simulink model "Parim_for_ai"  (R2024b)
settings: Solver=FixedStepDiscrete  StartTime=0.0  StopTime=3  FixedStep=Ts  RelTol=1e-3
PreLoadFcn:
  | Net_improve_init;L=Lac_MV;Tctrl=Ts;
PostLoadFcn:
  | Net_improve_init;L=Lac_MV;Tctrl=Ts;
InitFcn:
  | Net_improve_init;L=Lac_MV;Tctrl=Ts;
values from neighbouring files (symbols this model uses):
  Ts = 20e-6    (= 2e-05)    [Parsim_for_ai.m]
undefined symbols (not defined in the file or in its folder): C1, dend, DiscIntNeverNeededParam, fs, Lac_MV, numd, Pref, R1, Rac_MV, Vac_peak_MV, Vdc
libraries: powerlib_extras x10, spsControlledVoltageSourceLib x8, spsVoltageMeasurementLib x7, spsCurrentMeasurementLib x6, spsGroundLib x6, spsSeriesRLCBranchLib x6, spsACVoltageSourceLib x6, spsThreePhaseVIMeasurementLib x4, spsIdealSwitchLib x2, spsPower3phInstantaneousLib x2, simulink x2, spsThreePhaseSeriesRLCBranchLib x2
(part 1 of 2)
Description:
  | The Model initialization function Callback automatically
  | 
  | sets the sample time  to 2e-6 sec.  and loads the initial
  | 
  | states vector xInitial. The initial state vector is saved in the
  | 
  | power_acdrive_init.mat file.
  | 
  | 
  | 
  | Check  the Initial state checkbox in the Simulation
  | 
  | parameters/Workspace I/O to start in steady state with a
  | 
  | speed of 120 rad/s and a torque of 0 N.m/s,
  | 
  | 
  | Copyright 2008-2015 The MathWorks, Inc.
settings Model: Creator=WeiLi  LastModifiedBy=KeXing
settings SolverCC: AlgebraicLoopSolver=TrustRegion
settings DataIOCC: SaveFinalState=on  SaveFormat=Array  SignalLoggingSaveFormat=ModelDataLogs  SaveOutput=off  SaveTime=off  ReturnWorkspaceOutputs=off  SignalLoggingName=sigsOut
settings OptimizationCC: BlockReduction=off  ExpressionDepthLimit=2147483647  InitFltsAndDblsToZero=on  LifeSpan=inf
settings DebuggingCC: SaveWithParameterizedLinksMsg=none  UnderspecifiedInitializationDetection=Classic  MergeDetectMultiDrivingBlocksExec=none  CheckExecutionContextPreStartOutputMsg=on  SignalResolutionControl=TryResolveAllWithWarning  MultiTaskDSMMsg=warning  MultiTaskCondExecSysMsg=none  FcnCallInpInsideContextMsg=warning  UnconnectedInputMsg=warning  UnconnectedLineMsg=warning  StateNameClashWarn=warning  SFUnexpectedBacktrackingDiag=warning  SFNoUnconditionalDefaultTransitionDiag=warning  SFExecutionAtInitializationDiag=none  ArithmeticOperatorsInVariantConditions=warning
settings HardwareCC: ProdBitPerPointer=32  ProdBitPerSizeT=32  ProdBitPerPtrDiffT=32  ProdLargestAtomicFloat=None  ProdIntDivRoundTo=Undefined  ProdEndianess=Unspecified  ProdWordSize=32  ProdHWDeviceType=32-bit Generic  TargetUnknown=on
settings ModelReferenceCC: EnableRefExpFcnMdlSchedulingChecks=on  PropagateSignalLabelsOutOfModel=off
settings SFSimCC: SimUseLocalCustomCode=off  CustomCodeUndefinedFunction=UseInterfaceOnly
settings RTWCC: RTWUseLocalCustomCode=off  GPUComputeCapability=3.5
settings CodeAppCC: StateflowObjectComments=on
settings GRTTargetCC: TargetFcnLib=ansi_tfl_tmw.mat  TargetLangStandard=C89/C90 (ANSI)  CombineOutputUpdateFcns=off  GRTInterface=on
settings ConfigComp: CovMetricSettings=dw  CovSaveCumulativeToWorkspaceVar=on  CovSaveSingleToWorkspaceVar=on  CovExternalEMLEnable=off
settings SimscapeCC: SimscapeNormalizeSystem=off

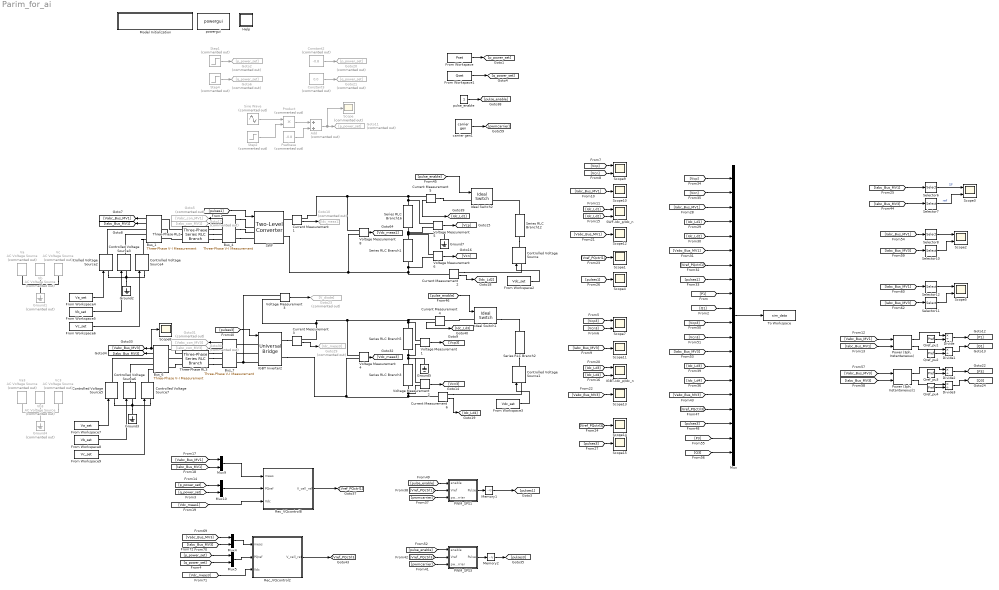
== system Parim_for_ai ==
  Add : Sum  Commented=on
  Bus_{1,4,6..7} (4 alike) : spsThreePhaseVIMeasurementLib/Three-Phase V-I Measurement  VoltageMeasurement=phase-to-ground  SetLabelV=off  LabelV=Vabc  Vpu=off  VpuLL=off  CurrentMeasurement=yes  SetLabelI=off  LabelI=Iabc  Ipu=off  Pbase=P_AC  Vbase=V_AC_prim  OutputType=Complex  PhasorSimulation=off  PSBequivalent=0
  Constant2 : Constant  Commented=on  Value=-0.8
  Constant3 : Constant  Commented=on  Value=0.0
  Controlled Voltage Source : spsControlledVoltageSourceLib/Controlled Voltage Source  Initialize=on  Source_Type=DC  Amplitude=3000  Phase=0  Frequency=0  Measurements=None
  Controlled Voltage Source1 : spsControlledVoltageSourceLib/Controlled Voltage Source  Initialize=on  Source_Type=DC  Amplitude=3000  Phase=0  Frequency=0  Measurements=None
  Controlled Voltage Source{2..7} (6 alike) : spsControlledVoltageSourceLib/Controlled Voltage Source  Initialize=off  Source_Type=AC  Amplitude=0  Phase=0  Frequency=fs  Measurements=None
  Current Measurement{1..6} (6 alike) : spsCurrentMeasurementLib/Current Measurement  PhasorSimulation=off  OutputType=Complex  PSBequivalent=0
  Divide{,1..3} (4 alike) : Product  Inputs=*/
  From Workspace : FromWorkspace  VariableName=Pset
  From Workspace1 : FromWorkspace  VariableName=Qset
  From Workspace2 : FromWorkspace  VariableName=Vdc_set  SampleTime=Ts
  From Workspace3 : FromWorkspace  VariableName=Vdc_set  SampleTime=Ts
  From Workspace4 : FromWorkspace  VariableName=Va_set  SampleTime=Ts
  From Workspace5 : FromWorkspace  VariableName=Vb_set  SampleTime=Ts
  From Workspace6 : FromWorkspace  VariableName=Vc_set  SampleTime=Ts
  From Workspace7 : FromWorkspace  VariableName=Va_set  SampleTime=Ts
  From Workspace8 : FromWorkspace  VariableName=Vb_set  SampleTime=Ts
  From Workspace9 : FromWorkspace  VariableName=Vc_set  SampleTime=Ts
  Goto10 : Goto  Commented=on  GotoTag=Idc_meas1
  Goto11 : Goto  Commented=on  GotoTag=p_power_set
  Goto17 : Goto  Commented=on  GotoTag=iabc_con_MV1
  Goto2 : Goto  Commented=on  GotoTag=p_power_set
  Goto20 : Goto  Commented=on  GotoTag=p_power_set
  Goto21 : Goto  Commented=on  GotoTag=q_power_set
  Goto23 : Goto  Commented=on  GotoTag=V_diode
  Goto29 : Goto  Commented=on  GotoTag=Idc_meas3
  Goto30 : Goto  Commented=on  GotoTag=iabc_con_MV3
  Goto31 : Goto  Commented=on  GotoTag=Vabc_con_MV3
  Goto5 : Goto  Commented=on  GotoTag=Vabc_con_MV1
  Goto6 : Goto  Commented=on  GotoTag=q_power_set
  Ground1 : spsGroundLib/Ground  Commented=on  LConnTagsString=a
  Ground{2..3,5,7} (4 alike) : spsGroundLib/Ground  LConnTagsString=a
  Ground4 : spsGroundLib/Ground  Commented=on  LConnTagsString=a
  Help : Subsystem  mask(OpDoc){docfile=../Help/help.html}
      mask init:
      | %patch([1,1,0,0,.8,1],[.8,0,0,1,1,.8],[.8 .8 .8]);
      | %patch([.15 .78 .78 .15 .15],[.8 .8 .83 .83 .8],[.9 .9 .9]);
      | %patch([.15 .78 .78 .15 .15],[.7 .7 .73 .73 .8],[.9 .9 .9]);
      | %patch([.15 .78 .78 .15 .15],[.6 .6 .63 .63 .6],[.9 .9 .9]);
      | %patch([.15 .78 .78 .15 .15],[.5 .5 .53 .53 .5],[.9 .9 .9]);
      | %patch([.15 .78 .78 .15 .15],[.4 .4 .43 .43 .4],[.9 .9 .9]);
      settings: OpenFcn=OpHelp_cb(gcb);
      mask Display: image(imread('opdoc.bmp'))
  IGBT Inverter2 : spsUniversalBridgeLib/Universal Bridge  Arms=3  SnubberResistance=IGBT_Rs  SnubberCapacitance=1e-6  Device=IGBT / Diodes  Ron=IGBT_Ron  Lon=0  ForwardVoltages=[0 0]  ForwardVoltage=.8  GTOparameters=[ 1e-6 , 1e-6 ]  IGBTparameters=[0 0]  Measurements=Device voltages  Measurements_2=None  converterType=Rectifier
      settings: AttributesFormatString=\n
  IGBT-Idc_p/Idc_n : Scope  NumInputPorts=2
  Ideal Switch1 : spsIdealSwitchLib/Ideal Switch  Ron=0.001  Lon=0  IC=0  Rs=1e9  Cs=inf  Measurements=on
  Ideal Switch2 : spsIdealSwitchLib/Ideal Switch  Ron=0.001  Lon=0  IC=0  Rs=1e9  Cs=inf  Measurements=on
  Memory1 : Memory
  Memory2 : Memory
  Model Initialization : Subsystem  mask(Model Functions){InitFcnX=Net_improve_init;L=Lac_MV;Tctrl=Ts;, prel=on, posl=on, inif=on, strf=off}
      mask prompts: InitFcnX "Initialisation"; prel "Preload Function"; posl "PostLoad Function"; inif "InitFcn"; strf "StartFcn"
      mask init:
      | currentBlock = gcb;
      | root = bdroot(currentBlock);
      | 
      | if ~strcmp(get_param(root,'BlockDiagramType'),'library')
      |     if prel==1
      |         set_param(root, 'PreLoadFcn', InitFcnX);
      |     else
      |         set_param(root, 'PreLoadFcn', '');
      |     end
      |     if inif==1
      |         set_param(root, 'InitFcn', InitFcnX);
      |     else
      |         set_param(root, 'InitFcn', '');
      |     end
      |     if strf==1
      |         set_param(root, 'StartFcn', InitFcnX);
      |     else
      |         set_param(root, 'StartFcn', '');
      |     end
      |     if posl==1
      |         set_param(root, 'PostLoadFcn', InitFcnX);
      |     else
      |         set_param(root, 'PostLoadFcn', '');
      |     end
      | end
      | 
      | pos = get_param(currentBlock, 'Position');
      | width = pos(3) - pos(1); height = pos(4) - pos(2);
      | txt = [ upper(root) '\n' '- InitFcn. . . . . '  get_param(root, 'InitFcn') ];
      settings: CopyFcn=set_param(gcb,'LinkStatus','none')
      mask Display: text(5, height*0.5, txt, 'horizontalAlignment', 'left', 'verticalAlignment', 'middle') ;
  Mux : Mux  Inputs=20
  Mux{4..5,9..10} (4 alike) : Mux  Inputs=2
  PWM_SPS1 : Subsystem
  PWM_SPS3 : Subsystem
  "Power (3ph, Instantaneous)" : spsPower3phInstantaneousLib/Power (3ph, Instantaneous)
  "Power (3ph, Instantaneous)1" : spsPower3phInstantaneousLib/Power (3ph, Instantaneous)
  Product : Product  Commented=on
  Psetbase : Constant  Commented=on  Value=-0.8
  Qref_pu{1..4} (4 alike) : Constant  Value=Pref
  Rec_VQcontrol2 : Subsystem  mask(converter controller){cm=off, base=[Pref, Vac_peak_MV*sqrt(3/2), Vdc/2, fs], LRx=[Lac_MV, Rac_MV], LRx_inpu=off, Kd=[0.3  2]*10/6  %was [1 0.1]   ; [0.1  1]*1, Kp=[0.3 1]*1     %was [1 0.1]   ; [0.1  1]*1, Kvdc=[2 10]*1;   %was [0.5 1]*20 for Cdc=320uF, Vabc_lim=[-1 1], limitVdq=1.1, nadv=6, xtrIctrl1=[0.4 10 10 -10], Ts=Tctrl}
      mask prompts: cm "control mode (check VQ/uncheck PQ), only one terminal in VQ mode"; base "base value for power(VA), ac voltage(V), dc voltage to ground(V), and frequenvy(Hz) [Sb, Vb, Vdcb,freq]"; LRx "commutation inductance and resistance [Lx, Rx]"; LRx_inpu "[Lx, Rx] in pu if checked/ SI unchecked"; Kd "Kp Ki for d-axis PI control [kp ki]"; Kp "Kp Ki for q-axis PI control [kp ki]"; Kvdc "Kp Ki for Vdc PI control [kp ki]"; Vabc_lim "output Vabc limit [min max]"; limitVdq "limit for Vd,Vq (pu, default = 1.1)"; nadv "nb of time step to compesate for delay (default=1)"; xtrIctrl1 "[kp, kp, limitmax, limitmin] for current control (default=[0.4, 10, 10, -10])"
      mask help:
      | input 1, 6 dimentions, Vabc, Iabc, (SI)
      | input 2, 2 dimentions, Pref, Qref (PU)
      | input 3, 6 dimentions, Vcap at up arm a, lower arm a, up arm b, lower arm b, up arm c and lower arm c.
      | input 4, 1 dimention, pulse on
      | input 5, 1 dimention
      |
      | power or current directions: to go into grid is positive
      mask init:
      | if cm==0;
      |     x=['PQ\nmode'];
      | else
      |     x=['VQ\nmode'];
      | end
      | 
      | Sb=base(1);            %VA 3phase power base;
      | Vb=base(2);       %V, line-line rms voltage base
      | Ib=Sb/(sqrt(3)*Vb); %A, rms current base
      | Zb=Vb^2/Sb ;        %ohm, impedence base
      | Vdc=base(3);      %V Vdc+ to ground or ground to Vdc- 
      | frq=base(4);
      | 
      | if LRx_inpu
      |     Rxpu=LRx(2);
      |     Lxpu=LRx(1);
      | else
      |     Rxpu=LRx(2)/Zb;
      |     Lxpu=LRx(1)*2*pi*frq/Zb;
      | end;
      | 
      | ks=Vdc*sqrt(3/2)/Vb;     % ma=1/ks for 1pu dc ->1pu ac;
      | 
      | Kp=Kd;
      mask DialogControl ParameterTabVar0 Prompt: parameters
      mask DialogControl ParameterTabVar01 Prompt: advanced
      mask Display: disp (x);
  Rec_VQcontrol8 : Subsystem  mask(converter controller){cm=off, base=[Pref, Vac_peak_MV*sqrt(3/2), Vdc/2, fs], LRx=[Lac_MV, Rac_MV], LRx_inpu=off, Kd=[0.3  2]*10/6  %was [1 0.1]   ; [0.1  1]*1, Kp=[0.3 1]*1     %was [1 0.1]   ; [0.1  1]*1, Kvdc=[2 10]*1;   %was [0.5 1]*20 for Cdc=320uF, Vabc_lim=[-1 1], limitVdq=1.1, nadv=6, xtrIctrl1=[0.4 10 10 -10], Ts=Tctrl}
      mask prompts: cm "control mode (check VQ/uncheck PQ), only one terminal in VQ mode"; base "base value for power(VA), ac voltage(V), dc voltage to ground(V), and frequenvy(Hz) [Sb, Vb, Vdcb,freq]"; LRx "commutation inductance and resistance [Lx, Rx]"; LRx_inpu "[Lx, Rx] in pu if checked/ SI unchecked"; Kd "Kp Ki for d-axis PI control [kp ki]"; Kp "Kp Ki for q-axis PI control [kp ki]"; Kvdc "Kp Ki for Vdc PI control [kp ki]"; Vabc_lim "output Vabc limit [min max]"; limitVdq "limit for Vd,Vq (pu, default = 1.1)"; nadv "nb of time step to compesate for delay (default=1)"; xtrIctrl1 "[kp, kp, limitmax, limitmin] for current control (default=[0.4, 10, 10, -10])"
      mask help:
      | input 1, 6 dimentions, Vabc, Iabc, (SI)
      | input 2, 2 dimentions, Pref, Qref (PU)
      | input 3, 6 dimentions, Vcap at up arm a, lower arm a, up arm b, lower arm b, up arm c and lower arm c.
      | input 4, 1 dimention, pulse on
      | input 5, 1 dimention
      |
      | power or current directions: to go into grid is positive
      mask init: same as Parim_for_ai/Rec_VQcontrol2
      mask DialogControl ParameterTabVar0 Prompt: parameters
      mask DialogControl ParameterTabVar01 Prompt: advanced
      mask Display: disp (x);
  SWF : spsTwoLevelConverterLib/Two-Level Converter  ModelType=Switching function  Ron=1e-3  Rs=1e6  Cs=inf  Vforward=[0,0]  Ron_Diode=IGBT_Ron  Rs_Diode=IGBT_Rs  Cs_Diode=1e-6  Vf_Diode=0  Rs_CurrentSource=inf  Ron_ACsource=1e-3
      settings: LibrarySourceBlock=sps_lib/Power Electronics/Two-Level Converter
  SWF-Idc_p/Idc_n : Scope  NumInputPorts=2
  Scope : Scope  Commented=on
  Scope{1,4,8,10..15} (9 alike) : Scope
  Scope{2..3,5,7,9} (5 alike) : Scope  NumInputPorts=2
  Selector10 : Selector  InputPortWidth=3  IndexOptions=Index vector (dialog)  Indices=[2]  OutputSizes=1
  Selector11 : Selector  InputPortWidth=3  IndexOptions=Index vector (dialog)  Indices=[3]  OutputSizes=1
  Selector12 : Selector  InputPortWidth=3  IndexOptions=Index vector (dialog)  Indices=[3]  OutputSizes=1
  Selector6 : Selector  InputPortWidth=3  IndexOptions=Index vector (dialog)  Indices=[1]  OutputSizes=1
  Selector7 : Selector  InputPortWidth=3  IndexOptions=Index vector (dialog)  Indices=[1]  OutputSizes=1
  Selector8 : Selector  InputPortWidth=3  IndexOptions=Index vector (dialog)  Indices=[2]  OutputSizes=1
  Series RLC Branch{1,3,5,16} (4 alike) : spsSeriesRLCBranchLib/Series RLC Branch  LConnTagsString=__new0  RConnTagsString=__new0  BranchType=C  Resistance=R1  Inductance=1e-3  SetiL0=off  InitialCurrent=0  Capacitance=C1  Setx0=off  InitialVoltage=0  Measurements=None
  Series RLC Branch12 : spsSeriesRLCBranchLib/Series RLC Branch  LConnTagsString=__new0  RConnTagsString=__new0  BranchType=R  Resistance=Vdc^2/(Pref)/10*2  Inductance=1e-3  SetiL0=off  InitialCurrent=0  Capacitance=C1  Setx0=off  InitialVoltage=0  Measurements=None
  Series RLC Branch2 : spsSeriesRLCBranchLib/Series RLC Branch  LConnTagsString=__new0  RConnTagsString=__new0  BranchType=R  Resistance=Vdc^2/(Pref)/10*2  Inductance=1e-3  SetiL0=off  InitialCurrent=0  Capacitance=C1  Setx0=off  InitialVoltage=0  Measurements=None
  Sine Wave : Sin  Commented=on  Amplitude=0.2  Frequency=20*2*pi  SampleTime=0
  Step1 : Step  Commented=on  Time=2  Before=-0.8  After=-0.5  SampleTime=0
  Step2 : Step  Commented=on  SampleTime=0
  Step4 : Step  Commented=on  Time=1.5  Before=0.0  After=0.0  SampleTime=0
  Three-Phase RL2 : spsThreePhaseSeriesRLCBranchLib/Three-Phase Series RLC Branch  LConnTagsString=A|B|C  RConnTagsString=A|B|C  BranchType=RL  Resistance=Rac_MV  Inductance=Lac_MV  Capacitance=1e-6  Measurements=None
  Three-Phase RL3 : spsThreePhaseSeriesRLCBranchLib/Three-Phase Series RLC Branch  LConnTagsString=A|B|C  RConnTagsString=A|B|C  BranchType=RL  Resistance=Rac_MV  Inductance=Lac_MV  Capacitance=1e-6  Measurements=None
  To Workspace : ToWorkspace  VariableName=sim_data  SampleTime=-1
      settings: Save2DSignal=2-D array (concatenate along first dimension)
  Va : spsACVoltageSourceLib/AC Voltage Source  Commented=on  Amplitude=Vac_peak_MV  Phase=0  Frequency=fs  SampleTime=Ts  Measurements=None  BusType=swing  Pref=10e3  Qref=0  Qmin=-inf  Qmax=+inf
  Va3 : spsACVoltageSourceLib/AC Voltage Source  Commented=on  Amplitude=Vac_peak_MV  Phase=0  Frequency=fs  SampleTime=Ts  Measurements=None  BusType=swing  Pref=10e3  Qref=0  Qmin=-inf  Qmax=+inf
  Vb : spsACVoltageSourceLib/AC Voltage Source  Commented=on  Amplitude=Vac_peak_MV  Phase=-120  Frequency=fs  SampleTime=Ts  Measurements=None  BusType=swing  Pref=10e3  Qref=0  Qmin=-inf  Qmax=+inf
  Vb3 : spsACVoltageSourceLib/AC Voltage Source  Commented=on  Amplitude=Vac_peak_MV  Phase=-120  Frequency=fs  SampleTime=Ts  Measurements=None  BusType=swing  Pref=10e3  Qref=0  Qmin=-inf  Qmax=+inf
  Vc : spsACVoltageSourceLib/AC Voltage Source  Commented=on  Amplitude=Vac_peak_MV  Phase=120  Frequency=fs  SampleTime=Ts  Measurements=None  BusType=swing  Pref=10e3  Qref=0  Qmin=-inf  Qmax=+inf
  Vc3 : spsACVoltageSourceLib/AC Voltage Source  Commented=on  Amplitude=Vac_peak_MV  Phase=120  Frequency=fs  SampleTime=Ts  Measurements=None  BusType=swing  Pref=10e3  Qref=0  Qmin=-inf  Qmax=+inf
  Voltage Measurement{1..6,8} (7 alike) : spsVoltageMeasurementLib/Voltage Measurement  PhasorSimulation=off  OutputType=Complex  PSBequivalent=0
  carrier gen1 : libMMCcpuv2/carrier gen  fc=f_cari  range=[ 1 -1]  Ms=3  Ns=1
  powergui : spspowerguiLib/powergui  Priority=2  SimulationMode=Discrete  SampleTime=Ts  frequency=60  Iterations=50  frequencyindice=0  Pbase=100e6  ErrMax=1e-4  UnitsV=kV  UnitsW=MW  buscounter=0  FunctionMessages=off  echomessages=off  EnableUseOfTLC=off  CurrentSourceSwitches=off  DisableSnubberDevices=off  DisableRonSwitches=off  DisableVfSwitches=off  DisplayEquations=off  AutomaticDiscreteSolvers=off  SolverType=Backward Euler  Interpol=off  ExternalGateDelay=off  methode=off  Ts=0  x0status=blocks  SPID=off  SwTol=0  HookPort=off  NonlinearTolerance=1e-4  nMaxIteration=100  ContinueOnMaxIteration=off  RestoreLinks=warning  ResistiveCurrentMeasurement=off  Frange=[0:2:500]  Ylog=off  Xlog=on  ShowGrid=off  save=off  variable=ZData  structure=VI  ZoomFFT=off  StartTime=9  cycles=10  DisplayStyle=2  fundamental=300/pi  FreqAxis=off  MaxFrequency=1000  frequencyindicesteady=1  RmsSteady=1  display=off
  pulse_enable : Constant
  wires:
  Bus_1/1 -> [Vabc_Bus_MV1]
  Bus_1/2 -> [Iabc_Bus_MV1]
  Bus_4/1 -> Goto5/1
  Current Measurement1/1 -> Goto10/1
  [Vabc_Bus_MV1] -> Mux9/1
  [Iabc_Bus_MV1] -> Mux9/2
  [q_power_set] -> Mux10/2
  carrier gen1/1 -> [pwmcarrier]
  [p_power_set] -> Mux10/1
  [pwmcarrier] -> PWM_SPS1/3(pwmcarrier)
  [Vref_PQctrl1] -> PWM_SPS1/2(Vref)
  Mux9/1 -> Rec_VQcontrol8/1(meas)
  Mux10/1 -> Rec_VQcontrol8/2(PQref)
  [Vdc_meas1] -> Rec_VQcontrol8/3(Vdc)
  Voltage Measurement8/1 -> [Vdc_meas1]
  Bus_4/2 -> Goto17/1
  [Iabc_Bus_MV1] -> Selector6/1
  Step2/1 -> Product/2
  Voltage Measurement3/1 -> Goto23/1
  Bus_6/1 -> Scope8/1, [Vabc_Bus_MV3]
  Bus_6/2 -> [Iabc_Bus_MV3]
  Bus_7/1 -> Goto31/1
  Current Measurement3/1 -> Goto29/1
  Voltage Measurement4/1 -> [Vdc_meas3]
  Bus_7/2 -> Goto30/1
  [pwmcarrier] -> PWM_SPS3/3(pwmcarrier)
  [Vref_PQctrl3] -> PWM_SPS3/2(Vref)
  [Iabc_Bus_MV3] -> Selector7/1
  [pulse_enable] -> PWM_SPS1/1(enable)
  [pulse_enable] -> PWM_SPS3/1(enable)
  Current Measurement5/1 -> [Idc_Ld1]
  Current Measurement4/1 -> [Idc_Ld3]
  [pulses3] -> IGBT Inverter2/1
  Selector6/1 -> Scope3/1  "SF"
  Selector7/1 -> Scope3/2  "ref"
  [Iabc_Bus_MV1] -> Selector8/1
  [Iabc_Bus_MV3] -> Selector10/1
  Selector8/1 -> Scope2/1
  Selector10/1 -> Scope2/2
  [Iabc_Bus_MV1] -> Selector12/1
  [Iabc_Bus_MV3] -> Selector11/1
  Selector12/1 -> Scope5/1
  Selector11/1 -> Scope5/2
  PWM_SPS1/1(Pulse) -> Memory1/1
  [Vabc_Bus_MV3] -> Mux4/1
  [Iabc_Bus_MV3] -> Mux4/2
  Mux4/1 -> Rec_VQcontrol2/1(meas)
  Mux5/1 -> Rec_VQcontrol2/2(PQref)
  [q_power_set] -> Mux5/2
  [Vdc_meas3] -> Rec_VQcontrol2/3(Vdc)
  [p_power_set] -> Mux5/1
  [pulse_enable] -> Ideal Switch2/1
  [pulse_enable] -> Ideal Switch1/1
  Memory1/1 -> [pulses1]
  pulse_enable/1 -> [pulse_enable]
  PWM_SPS3/1(Pulse) -> Memory2/1
  Rec_VQcontrol8/1(V_cell_ref) -> [Vref_PQctrl1]
  Rec_VQcontrol2/1(V_cell_ref) -> [Vref_PQctrl3]
  Memory2/1 -> [pulses3]
  "Power (3ph, Instantaneous)"/1 -> Divide/1
  Qref_pu2/1 -> Divide1/2
  [Iabc_Bus_MV1] -> "Power (3ph, Instantaneous)"/2
  Divide1/1 -> [Q1]
  Qref_pu1/1 -> Divide/2
  Divide/1 -> [P1]
  [Vabc_Bus_MV1] -> "Power (3ph, Instantaneous)"/1
  "Power (3ph, Instantaneous)"/2 -> Divide1/1
  From Workspace1/1 -> [q_power_set]
  Step1/1 -> Goto2/1
  Product/1 -> Add/1
  Psetbase/1 -> Add/2
  Add/1 -> Scope/1, Goto11/1
  Sine Wave/1 -> Product/1
  From Workspace/1 -> [p_power_set]
  Step4/1 -> Goto6/1
  Voltage Measurement1/1 -> [Vcp3]
  Voltage Measurement2/1 -> [Vcn3]
  [Vcp3] -> Scope7/1
  [Vcn3] -> Scope7/2
  Voltage Measurement5/1 -> [Vcp]
  Voltage Measurement6/1 -> [Vcn]
  [Vcp] -> Scope9/1
  [Vcn] -> Scope9/2
  [Iabc_Bus_MV1] -> Scope10/1
  [Iabc_Bus_MV3] -> Scope11/1
  Current Measurement2/1 -> [Idc_Ld2]
  Current Measurement6/1 -> [Idc_Ld4]
  [Idc_Ld1] -> SWF-Idc_p/Idc_n/1
  [Idc_Ld2] -> SWF-Idc_p/Idc_n/2
  [Idc_Ld3] -> IGBT-Idc_p/Idc_n/1
  [Idc_Ld4] -> IGBT-Idc_p/Idc_n/2
  [Vabc_Bus_MV1] -> Scope12/1
  [Vabc_Bus_MV3] -> Scope13/1
  [Vref_PQctrl1] -> Scope1/1
  [pulses1] -> Scope4/1
  [Vref_PQctrl3] -> Scope14/1
  [pulses3] -> Scope15/1
  Constant2/1 -> Goto20/1
  Constant3/1 -> Goto21/1
  [Vcp] -> Mux/1
  [Vcn] -> Mux/2
  [Iabc_Bus_MV1] -> Mux/3
  [Idc_Ld1] -> Mux/4
  [Idc_Ld2] -> Mux/5
  [Vabc_Bus_MV1] -> Mux/6
  [Vref_PQctrl1] -> Mux/7
  [pulses1] -> Mux/8
  Mux/1 -> To Workspace/1
  From Workspace2/1 -> Controlled Voltage Source/1
  From Workspace3/1 -> Controlled Voltage Source1/1
  [P1] -> Mux/9
  [Q1] -> Mux/10
  [pulses3] -> Mux/18
  [Iabc_Bus_MV3] -> Mux/13
  [Idc_Ld4] -> Mux/15
  [Vcp3] -> Mux/11
  [Idc_Ld3] -> Mux/14
  [Vref_PQctrl3] -> Mux/17
  [Vcn3] -> Mux/12
  [Vabc_Bus_MV3] -> Mux/16
  "Power (3ph, Instantaneous)1"/1 -> Divide2/1
  Qref_pu3/1 -> Divide2/2
  Divide3/1 -> [Q3]
  "Power (3ph, Instantaneous)1"/2 -> Divide3/1
  Qref_pu4/1 -> Divide3/2
  Divide2/1 -> [P3]
  [Iabc_Bus_MV3] -> "Power (3ph, Instantaneous)1"/2
  [Vabc_Bus_MV3] -> "Power (3ph, Instantaneous)1"/1
  [Q3] -> Mux/20
  [P3] -> Mux/19
  From Workspace4/1 -> Controlled Voltage Source2/1
  From Workspace5/1 -> Controlled Voltage Source3/1
  From Workspace6/1 -> Controlled Voltage Source4/1
  [pulses1] -> SWF/1
  From Workspace7/1 -> Controlled Voltage Source5/1
  From Workspace8/1 -> Controlled Voltage Source6/1
  From Workspace9/1 -> Controlled Voltage Source7/1
  connections:
  Three-Phase RL2/LConn1 -- Bus_1/LConn1
  Three-Phase RL2/LConn3 -- Bus_1/LConn3
  Three-Phase RL2/LConn2 -- Bus_1/LConn2
  Three-Phase RL2/RConn1 -- Bus_4/RConn1
  Three-Phase RL2/RConn2 -- Bus_4/RConn2
  Three-Phase RL2/RConn3 -- Bus_4/RConn3
  Series RLC Branch1/RConn1 -- Voltage Measurement6/LConn2 -- Current Measurement2/LConn1 -- Voltage Measurement8/LConn2 -- SWF/RConn2
  Voltage Measurement8/LConn1 -- Current Measurement5/RConn1 -- Voltage Measurement5/LConn1 -- Series RLC Branch16/LConn1 -- Current Measurement1/RConn1
  Series RLC Branch1/LConn1 -- Voltage Measurement6/LConn1 -- Ground7/LConn1 -- Voltage Measurement5/LConn2 -- Series RLC Branch16/RConn1
  IGBT Inverter2/LConn1 -- Bus_7/LConn1
  Series RLC Branch3/RConn1 -- Voltage Measurement2/LConn2 -- Current Measurement6/LConn1 -- IGBT Inverter2/RConn2 -- Voltage Measurement4/LConn2
  Series RLC Branch5/LConn1 -- Voltage Measurement1/LConn1 -- Current Measurement4/RConn1 -- Voltage Measurement4/LConn1 -- Voltage Measurement3/LConn2 -- Current Measurement3/RConn1
  Series RLC Branch3/LConn1 -- Voltage Measurement2/LConn1 -- Ground5/LConn1 -- Voltage Measurement1/LConn2 -- Series RLC Branch5/RConn1
  IGBT Inverter2/RConn1 -- Current Measurement3/LConn1
  Three-Phase RL3/RConn1 -- Bus_7/RConn1
  Bus_6/RConn2 -- Controlled Voltage Source6/RConn1
  Three-Phase RL3/LConn2 -- Bus_6/LConn2
  Bus_6/RConn3 -- Controlled Voltage Source7/RConn1
  Three-Phase RL3/RConn3 -- Bus_7/RConn3
  Three-Phase RL3/RConn2 -- Bus_7/RConn2
  Three-Phase RL3/LConn3 -- Bus_6/LConn3
  Bus_6/RConn1 -- Controlled Voltage Source5/RConn1
  Three-Phase RL3/LConn1 -- Bus_6/LConn1
  IGBT Inverter2/LConn3 -- Voltage Measurement3/LConn1 -- Bus_7/LConn3
  IGBT Inverter2/LConn2 -- Bus_7/LConn2
  Ideal Switch1/RConn1 -- Series RLC Branch2/RConn1
  Current Measurement5/LConn1 -- Ideal Switch2/LConn1
  Series RLC Branch2/LConn1 -- Controlled Voltage Source1/RConn1
  Series RLC Branch12/LConn1 -- Controlled Voltage Source/RConn1
  Series RLC Branch12/RConn1 -- Ideal Switch2/RConn1
  Current Measurement2/RConn1 -- Controlled Voltage Source/LConn1
  Current Measurement6/RConn1 -- Controlled Voltage Source1/LConn1
  Vb3/LConn1 -- Vc3/LConn1 -- Va3/LConn1 -- Ground4/LConn1
  Ground1/LConn1 -- Vb/LConn1 -- Vc/LConn1 -- Va/LConn1
  Ground2/LConn1 -- Controlled Voltage Source4/LConn1 -- Controlled Voltage Source2/LConn1 -- Controlled Voltage Source3/LConn1
  Ground3/LConn1 -- Controlled Voltage Source7/LConn1 -- Controlled Voltage Source5/LConn1 -- Controlled Voltage Source6/LConn1
  Ideal Switch1/LConn1 -- Current Measurement4/LConn1
  Bus_1/RConn1 -- Controlled Voltage Source2/RConn1
  Bus_1/RConn2 -- Controlled Voltage Source3/RConn1
  Bus_1/RConn3 -- Controlled Voltage Source4/RConn1
  Current Measurement1/LConn1 -- SWF/RConn1
  Bus_4/LConn3 -- SWF/LConn3
  Bus_4/LConn2 -- SWF/LConn2
  Bus_4/LConn1 -- SWF/LConn1

== system Parim_for_ai/Help ==

== system Parim_for_ai/Model Initialization ==

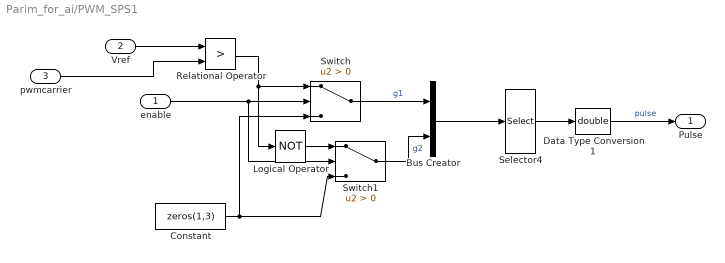
== system Parim_for_ai/PWM_SPS1 ==
  enable : Inport
  Vref : Inport  Port=2
  pwmcarrier : Inport  Port=3
  Bus Creator : BusCreator  Inputs=2
  Constant : Constant  Value=zeros(1,3)
  Data Type Conversion1 : DataTypeConversion  OutDataTypeStr=double  SaturateOnIntegerOverflow=off  RndMeth=Floor
  Logical Operator : Logic  Operator=NOT  AllPortsSameDT=off  OutDataTypeStr=boolean
  Relational Operator : RelationalOperator  Operator=>  OutDataTypeStr=boolean  InputSameDT=off
  Selector4 : Selector  InputPortWidth=6  IndexOptions=Index vector (dialog)  Indices=[1 4 2 5 3 6]  OutputSizes=1
  Switch : Switch  Criteria=u2 > Threshold  SaturateOnIntegerOverflow=off  InputSameDT=off
  Switch1 : Switch  Criteria=u2 > Threshold  SaturateOnIntegerOverflow=off  InputSameDT=off
  Pulse : Outport  VectorParamsAs1DForOutWhenUnconnected=off
  wires:
  Vref/1 -> Relational Operator/1
  pwmcarrier/1 -> Relational Operator/2
  enable/1 -> Switch1/2, Switch/2
  Relational Operator/1 -> Logical Operator/1, Switch/1
  Switch/1 -> Bus Creator/1  "g1"
  Switch1/1 -> Bus Creator/2  "g2"
  Logical Operator/1 -> Switch1/1
  Constant/1 -> Switch/3, Switch1/3
  Selector4/1 -> Data Type Conversion1/1
  Bus Creator/1 -> Selector4/1
  Data Type Conversion1/1 -> Pulse/1  "pulse"

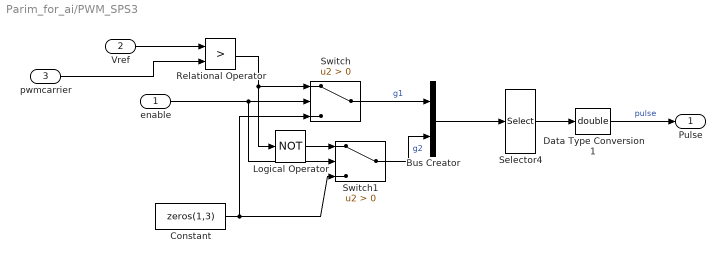
== system Parim_for_ai/PWM_SPS3 ==
  enable : Inport
  Vref : Inport  Port=2
  pwmcarrier : Inport  Port=3
  Bus Creator : BusCreator  Inputs=2
  Constant : Constant  Value=zeros(1,3)
  Data Type Conversion1 : DataTypeConversion  OutDataTypeStr=double  SaturateOnIntegerOverflow=off  RndMeth=Floor
  Logical Operator : Logic  Operator=NOT  AllPortsSameDT=off  OutDataTypeStr=boolean
  Relational Operator : RelationalOperator  Operator=>  OutDataTypeStr=boolean  InputSameDT=off
  Selector4 : Selector  InputPortWidth=6  IndexOptions=Index vector (dialog)  Indices=[1 4 2 5 3 6]  OutputSizes=1
  Switch : Switch  Criteria=u2 > Threshold  SaturateOnIntegerOverflow=off  InputSameDT=off
  Switch1 : Switch  Criteria=u2 > Threshold  SaturateOnIntegerOverflow=off  InputSameDT=off
  Pulse : Outport  VectorParamsAs1DForOutWhenUnconnected=off
  wires:
  Data Type Conversion1/1 -> Pulse/1  "pulse"
  Bus Creator/1 -> Selector4/1
  Selector4/1 -> Data Type Conversion1/1
  Constant/1 -> Switch1/3, Switch/3
  Logical Operator/1 -> Switch1/1
  Switch1/1 -> Bus Creator/2  "g2"
  Switch/1 -> Bus Creator/1  "g1"
  Relational Operator/1 -> Switch/1, Logical Operator/1
  enable/1 -> Switch/2, Switch1/2
  pwmcarrier/1 -> Relational Operator/2
  Vref/1 -> Relational Operator/1

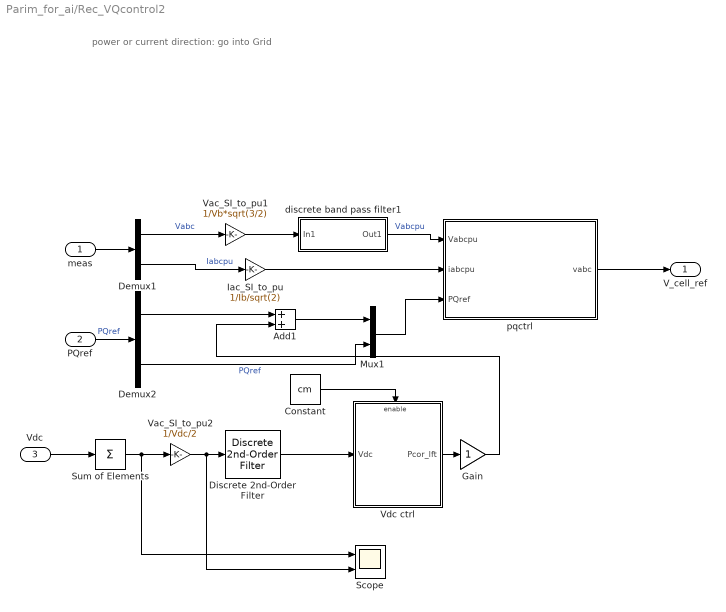
== system Parim_for_ai/Rec_VQcontrol2 ==
  note: power or current direction: go into Grid
  meas : Inport
  PQref : Inport  Port=2
  Vdc : Inport  Port=3
  Add1 : Sum
  Constant : Constant  Value=cm
  Demux1 : Demux  Outputs=[3 3 ]
  Demux2 : Demux  Outputs=2
  Discrete 2nd-Order Filter : powerlib_extras/Discrete  Control Blocks/Discrete  2nd-Order Filter  FilterType=Lowpass  Fo=90  Zeta=0.707  Ts=Ts  Initialize=off  Vac_Init=[0.8 -25 60]  Vdc_Init=-0.4  PlotResponse=off  param1=[1 500 1]
  Gain : Gain
  Iac_SI_to_pu : Gain  Gain=1/Ib/sqrt(2)
  Mux1 : Mux  Inputs=2
  Scope : Scope  NumInputPorts=2
  Sum of Elements : Sum  Inputs=+
  Vac_SI_to_pu1 : Gain  Gain=1/Vb*sqrt(3/2)
  Vac_SI_to_pu2 : Gain  Gain=1/Vdc/2  SampleTime=Ts
  Vdc ctrl : Subsystem
  discrete band pass filter1 : Subsystem  mask(discrete transfer Fcn generator){Fo=frq, adj1=1, inistate=0, Ts=Ts, bodedw=off}
      mask prompts: Fo "F0 (Hz)"; adj1 "adj (1 for no adjustment, larger adj for wider band pass)"; inistate "Initial states"; Ts "Sample time (must be explicite)"; bodedw "draw Bode diagram of filter"
      mask help:
      | This block transfer a continous TF to a discrete TF
      | using Bilinear (Tustin) approximation
      mask init:
      | AD1=tf([1 0],1);
      | 
      | %second order
      | % Fo=50; %cut off freq.
      | % omega0=Fo*2*pi;
      | % adj1=3;   %adjustment 1
      | Zeta= 0.707*adj1; %Damping factor Zeta ( Q = 1 / (2*Zeta) ):
      | Wo=2*pi*Fo;
      | % str=sprintf(' Fo=%iHz\n\n',Fo);
      |  n2=0; n1=0;n0=Wo*Wo;
      |  d2=1;d1=2*Zeta*Wo;d0=Wo*Wo;
      | numc=[n2 n1 n0];
      | denc=[d2 d1 d0];
      | AD3=tf(numc,denc);
      | 
      | AD4=AD1*AD3;
      | [mag1,pha1]=bode(AD4,Wo);
      | mag0=mag1;
      | AD=AD4/mag0;
      | 
      | if bodedw==1
      |     figure;
      |     h=bodeplot(AD1,AD3,AD);
      |     setoptions(h,'FreqUnits','Hz');
      |     grid on;
      |     title(['Bode Diagram, adj=',num2str(adj1)]);
      | end;
      |     
      | % gg=tf(num,den);
      | ggd=c2d(AD,Ts,'tustin');
      | [numd,dend] = tfdata(ggd,'v');
  pqctrl : Subsystem
  V_cell_ref : Outport  VectorParamsAs1DForOutWhenUnconnected=off
  wires:
  Gain/1 -> Add1/2
  Sum of Elements/1 -> Vac_SI_to_pu2/1, Scope/1
  pqctrl/1(vabc) -> V_cell_ref/1
  PQref/1 -> Demux2/1  "PQref"
  discrete band pass filter1/1(Out1) -> pqctrl/1(Vabcpu)  "Vabcpu"
  meas/1 -> Demux1/1
  Demux1/2 -> Iac_SI_to_pu/1  "Iabcpu"
  Demux1/1 -> Vac_SI_to_pu1/1  "Vabc"
  Iac_SI_to_pu/1 -> pqctrl/2(iabcpu)
  Demux2/1 -> Add1/1
  Vdc ctrl/1(Pcor_lft) -> Gain/1
  Add1/1 -> Mux1/1
  Demux2/2 -> Mux1/2  "PQref"
  Mux1/1 -> pqctrl/3(PQref)
  Discrete 2nd-Order Filter/1 -> Vdc ctrl/1(Vdc)
  Vdc/1 -> Sum of Elements/1
  Vac_SI_to_pu2/1 -> Discrete 2nd-Order Filter/1, Scope/2
  Vac_SI_to_pu1/1 -> discrete band pass filter1/1(In1)
  Constant/1 -> Vdc ctrl/Enable

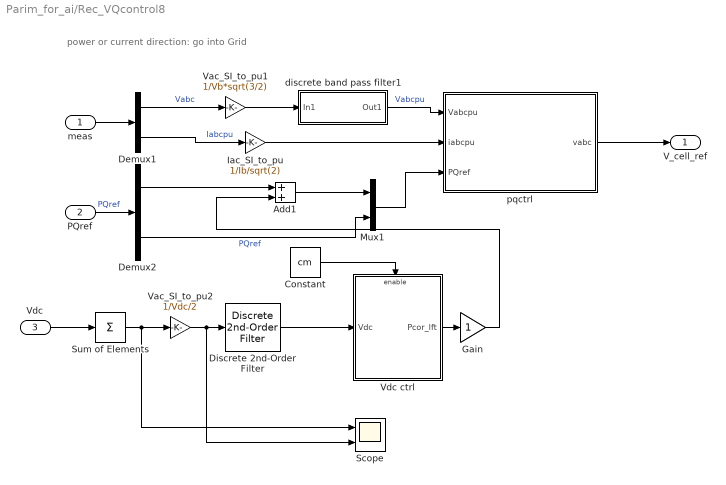
== system Parim_for_ai/Rec_VQcontrol8 ==
  note: power or current direction: go into Grid
  meas : Inport
  PQref : Inport  Port=2
  Vdc : Inport  Port=3
  Add1 : Sum
  Constant : Constant  Value=cm
  Demux1 : Demux  Outputs=[3 3 ]
  Demux2 : Demux  Outputs=2
  Discrete 2nd-Order Filter : powerlib_extras/Discrete  Control Blocks/Discrete  2nd-Order Filter  FilterType=Lowpass  Fo=90  Zeta=0.707  Ts=Ts  Initialize=off  Vac_Init=[0.8 -25 60]  Vdc_Init=-0.4  PlotResponse=off  param1=[1 500 1]
  Gain : Gain
  Iac_SI_to_pu : Gain  Gain=1/Ib/sqrt(2)
  Mux1 : Mux  Inputs=2
  Scope : Scope  NumInputPorts=2
  Sum of Elements : Sum  Inputs=+
  Vac_SI_to_pu1 : Gain  Gain=1/Vb*sqrt(3/2)
  Vac_SI_to_pu2 : Gain  Gain=1/Vdc/2  SampleTime=Ts
  Vdc ctrl : Subsystem
  discrete band pass filter1 : Subsystem  mask(discrete transfer Fcn generator){Fo=frq, adj1=1, inistate=0, Ts=Ts, bodedw=off}
      mask prompts: Fo "F0 (Hz)"; adj1 "adj (1 for no adjustment, larger adj for wider band pass)"; inistate "Initial states"; Ts "Sample time (must be explicite)"; bodedw "draw Bode diagram of filter"
      mask help:
      | This block transfer a continous TF to a discrete TF
      | using Bilinear (Tustin) approximation
      mask init: same as Parim_for_ai/Rec_VQcontrol2/discrete band pass filter1
  pqctrl : Subsystem
  V_cell_ref : Outport  VectorParamsAs1DForOutWhenUnconnected=off
  wires:
  Constant/1 -> Vdc ctrl/Enable
  Vac_SI_to_pu1/1 -> discrete band pass filter1/1(In1)
  Vac_SI_to_pu2/1 -> Scope/2, Discrete 2nd-Order Filter/1
  Vdc/1 -> Sum of Elements/1
  Discrete 2nd-Order Filter/1 -> Vdc ctrl/1(Vdc)
  Mux1/1 -> pqctrl/3(PQref)
  Demux2/2 -> Mux1/2  "PQref"
  Add1/1 -> Mux1/1
  Vdc ctrl/1(Pcor_lft) -> Gain/1
  Demux2/1 -> Add1/1
  Iac_SI_to_pu/1 -> pqctrl/2(iabcpu)
  Demux1/1 -> Vac_SI_to_pu1/1  "Vabc"
  Demux1/2 -> Iac_SI_to_pu/1  "Iabcpu"
  meas/1 -> Demux1/1
  discrete band pass filter1/1(Out1) -> pqctrl/1(Vabcpu)  "Vabcpu"
  PQref/1 -> Demux2/1  "PQref"
  pqctrl/1(vabc) -> V_cell_ref/1
  Sum of Elements/1 -> Scope/1, Vac_SI_to_pu2/1
  Gain/1 -> Add1/2

== system Parim_for_ai/Rec_VQcontrol2/Vdc ctrl ==
  Vdc : Inport
  Enable : EnablePort  StatesWhenEnabling=reset
  Vdc_ctrler1 : Subsystem
  Pcor_lft : Outport  OutputWhenDisabled=reset  InitialOutput=0  VectorParamsAs1DForOutWhenUnconnected=off
  wires:
  Vdc/1 -> Vdc_ctrler1/1(Vcap)
  Vdc_ctrler1/1(delP) -> Pcor_lft/1  "Pclft"

== system Parim_for_ai/Rec_VQcontrol2/discrete band pass filter1 ==
  In1 : Inport
  Discrete Transfer Fcn : DiscreteTransferFcn  Numerator=numd  Denominator=dend  InitialStates=inistate  SampleTime=Ts
  Out1 : Outport  VectorParamsAs1DForOutWhenUnconnected=off
  wires:
  In1/1 -> Discrete Transfer Fcn/1
  Discrete Transfer Fcn/1 -> Out1/1

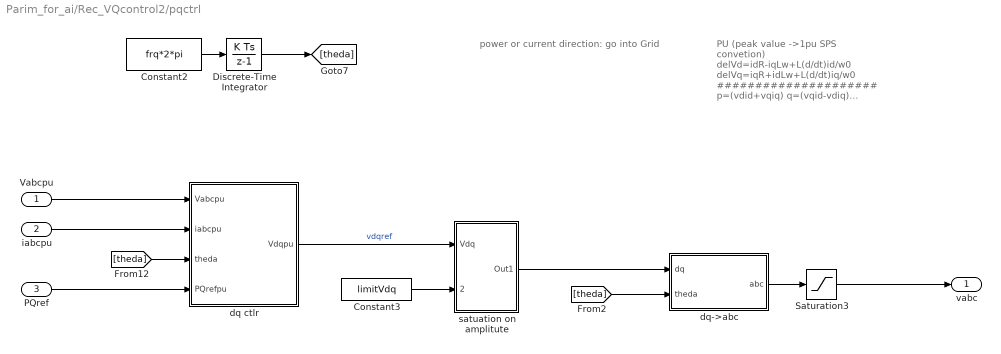
== system Parim_for_ai/Rec_VQcontrol2/pqctrl ==
  note: power or current direction: go into Grid
  note: PU
      | (peak value ->1pu
      | SPS convetion)
      |
      | delVd=idR-iqLw+L(d/dt)id/w0
      | delVq=iqR+idLw+L(d/dt)iq/w0
      | #####################
      | p=(vdid+vqiq)
      | q=(vqid-vdiq)
      | =>
      | Id=(Vd*P+Vq*Q)/C
      | Iq=(Vq*P-Vd*Q)/C
      | C=Vd^2+Vq^2
  Vabcpu : Inport
  iabcpu : Inport  Port=2
  PQref : Inport  Port=3
  Constant2 : Constant  Value=frq*2*pi
  Constant3 : Constant  Value=limitVdq
  Discrete-Time Integrator : DiscreteIntegrator  SampleTime=Ts  ICPrevOutput=DiscIntNeverNeededParam  ICPrevScaledInput=DiscIntNeverNeededParam
  Saturation3 : Saturate  UpperLimit=Vabc_lim(2)  LowerLimit=Vabc_lim(1)
  dq ctlr : Subsystem
  dq->abc : Subsystem
  "satuation on amplitute " : Subsystem
  vabc : Outport  VectorParamsAs1DForOutWhenUnconnected=off
  wires:
  PQref/1 -> dq ctlr/4(PQrefpu)
  iabcpu/1 -> dq ctlr/2(iabcpu)
  Vabcpu/1 -> dq ctlr/1(Vabcpu)
  dq ctlr/1(Vdqpu) -> "satuation on amplitute "/1(Vdq)  "vdqref"
  [theda] -> dq ctlr/3(theda)
  Discrete-Time Integrator/1 -> [theda]
  Constant2/1 -> Discrete-Time Integrator/1
  "satuation on amplitute "/1(Out1) -> dq->abc/1(dq)
  Constant3/1 -> "satuation on amplitute "/2(limitVdq)
  dq->abc/1(abc) -> Saturation3/1
  [theda] -> dq->abc/2(theda)
  Saturation3/1 -> vabc/1

== system Parim_for_ai/Rec_VQcontrol8/Vdc ctrl ==
  Vdc : Inport
  Enable : EnablePort  StatesWhenEnabling=reset
  Vdc_ctrler1 : Subsystem
  Pcor_lft : Outport  OutputWhenDisabled=reset  InitialOutput=0  VectorParamsAs1DForOutWhenUnconnected=off
  wires:
  Vdc_ctrler1/1(delP) -> Pcor_lft/1  "Pclft"
  Vdc/1 -> Vdc_ctrler1/1(Vcap)

== system Parim_for_ai/Rec_VQcontrol8/discrete band pass filter1 ==
  In1 : Inport
  Discrete Transfer Fcn : DiscreteTransferFcn  Numerator=numd  Denominator=dend  InitialStates=inistate  SampleTime=Ts
  Out1 : Outport  VectorParamsAs1DForOutWhenUnconnected=off
  wires:
  Discrete Transfer Fcn/1 -> Out1/1
  In1/1 -> Discrete Transfer Fcn/1

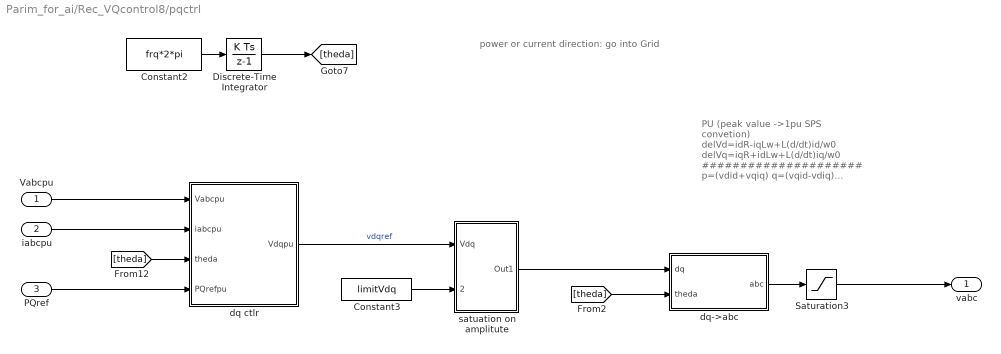
== system Parim_for_ai/Rec_VQcontrol8/pqctrl ==
  note: PU
      | (peak value ->1pu
      | SPS convetion)
      |
      | delVd=idR-iqLw+L(d/dt)id/w0
      | delVq=iqR+idLw+L(d/dt)iq/w0
      | #####################
      | p=(vdid+vqiq)
      | q=(vqid-vdiq)
      | =>
      | Id=(Vd*P+Vq*Q)/C
      | Iq=(Vq*P-Vd*Q)/C
      | C=Vd^2+Vq^2
  note: power or current direction: go into Grid
  Vabcpu : Inport
  iabcpu : Inport  Port=2
  PQref : Inport  Port=3
  Constant2 : Constant  Value=frq*2*pi
  Constant3 : Constant  Value=limitVdq
  Discrete-Time Integrator : DiscreteIntegrator  SampleTime=Ts  ICPrevOutput=DiscIntNeverNeededParam  ICPrevScaledInput=DiscIntNeverNeededParam
  Saturation3 : Saturate  UpperLimit=Vabc_lim(2)  LowerLimit=Vabc_lim(1)
  dq ctlr : Subsystem
  dq->abc : Subsystem
  "satuation on amplitute " : Subsystem
  vabc : Outport  VectorParamsAs1DForOutWhenUnconnected=off
  wires:
  Saturation3/1 -> vabc/1
  [theda] -> dq->abc/2(theda)
  dq->abc/1(abc) -> Saturation3/1
  Constant3/1 -> "satuation on amplitute "/2(limitVdq)
  "satuation on amplitute "/1(Out1) -> dq->abc/1(dq)
  Constant2/1 -> Discrete-Time Integrator/1
  Discrete-Time Integrator/1 -> [theda]
  [theda] -> dq ctlr/3(theda)
  dq ctlr/1(Vdqpu) -> "satuation on amplitute "/1(Vdq)  "vdqref"
  Vabcpu/1 -> dq ctlr/1(Vabcpu)
  iabcpu/1 -> dq ctlr/2(iabcpu)
  PQref/1 -> dq ctlr/4(PQrefpu)

== system Parim_for_ai/Rec_VQcontrol2/Vdc ctrl/Vdc_ctrler1 ==
  Vcap : Inport
  Add2 : Sum  Inputs=+-
  PI_d2 : Subsystem  AncestorBlock=|  DialogController=POWERSYS.PowerSysDialog  mask(Discrete PI Controller){Kp=Kvdc(1), Ki=Kvdc(2), Par_Limits=[1 -1]*1, Init=0, Ts=Ts}
      | powerlib_extras/Discrete 
      | Control Blocks/Discrete
      | PI Controller
      mask prompts: Kp "Proportional gain (Kp):"; Ki "Integral gain (Ki):"; Par_Limits "Output limits: [ Upper   Lower ]"; Init "Output initial value:"; Ts "Sample time:"
      mask help: This block implements a discrete PI controller.
      mask init:
      | UpperLimit=Par_Limits(1);
      | LowerLimit=Par_Limits(2);
      | power_initmask();
      mask Help: This block is part of a subset of blocks in the Extras library that does not have documentation associated with it, other than the block mask description.
      mask Display: disp('PI');
  Saturation : Saturate  UpperLimit=0.1  LowerLimit=-0.1
      settings: AttributesFormatString=%<LowerLimit>~%<UpperLimit>
  Vdcpuref : Constant
  Vdctrl : Scope  NumInputPorts=2
  delP : Outport  OutputWhenDisabled=reset  InitialOutput=[0]  VectorParamsAs1DForOutWhenUnconnected=off
  wires:
  Add2/1 -> Saturation/1  "delVdc"
  Vcap/1 -> Vdctrl/1, Add2/1
  Vdcpuref/1 -> Add2/2
  Saturation/1 -> PI_d2/1(Error)
  PI_d2/1(Out) -> Vdctrl/2, delP/1  "PIVdc"

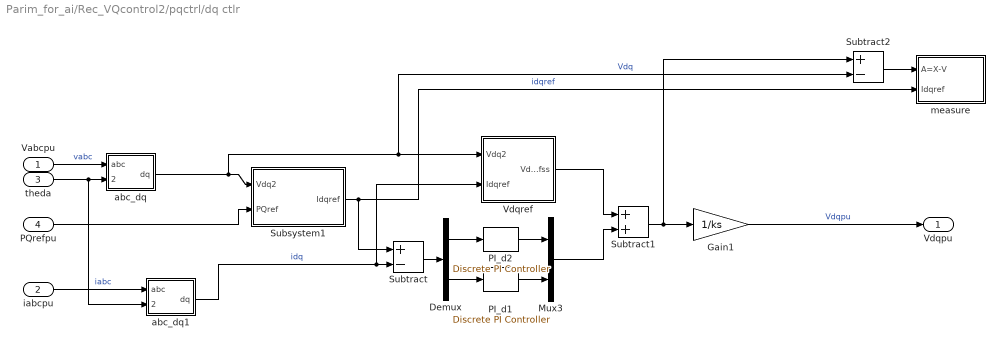
== system Parim_for_ai/Rec_VQcontrol2/pqctrl/dq ctlr ==
  Vabcpu : Inport
  iabcpu : Inport  Port=2
  theda : Inport  Port=3
  PQrefpu : Inport  Port=4
  Demux : Demux  Outputs=2
  Gain1 : Gain  Gain=1/ks
  Mux3 : Mux  Inputs=2
  PI_d1 : powerlib_extras/Discrete  Control Blocks/Discrete PI Controller  Kp=Kp(1)  Ki=Kp(2)  Par_Limits=[1 -1]*0.15  Init=0  Ts=Ts
  PI_d2 : powerlib_extras/Discrete  Control Blocks/Discrete PI Controller  Kp=Kd(1)  Ki=Kd(2)  Par_Limits=[1 -1]*0.25  Init=0  Ts=Ts
  Subsystem1 : Subsystem
  Subtract : Sum  Inputs=+-
  Subtract1 : Sum
  Subtract2 : Sum  Inputs=+-
  Vdqref : Subsystem
  abc_dq : Subsystem
  abc_dq1 : Subsystem
  measure : Subsystem
  Vdqpu : Outport  VectorParamsAs1DForOutWhenUnconnected=off
  wires:
  Gain1/1 -> Vdqpu/1  "Vdqpu"
  iabcpu/1 -> abc_dq1/1(abc)  "iabc"
  PQrefpu/1 -> Subsystem1/2(PQref)
  theda/1 -> abc_dq1/2(theta), abc_dq/2(theta)
  Vabcpu/1 -> abc_dq/1(abc)  "vabc"
  Subtract1/1 -> Gain1/1, Subtract2/1
  Mux3/1 -> Subtract1/2
  PI_d1/1 -> Mux3/2
  PI_d2/1 -> Mux3/1
  Vdqref/1(Vdqrefss) -> Subtract1/1
  Demux/2 -> PI_d1/1
  Demux/1 -> PI_d2/1
  Subtract/1 -> Demux/1
  abc_dq1/1(dq) -> Subtract/2, Vdqref/2(Idqref)  "idq"
  abc_dq/1(dq) -> Subsystem1/1(Vdq2), Vdqref/1(Vdq2), Subtract2/2  "Vdq"
  Subsystem1/1(Idqref) -> Subtract/1, measure/2(Idqref)  "idqref"
  Subtract2/1 -> measure/1(A=X-V)

== system Parim_for_ai/Rec_VQcontrol2/pqctrl/dq->abc ==
  note: Vc= Vd*sin(wt+2pi/3) + Vq*cos(wt+2pi/3) + Vo
  note: Vb= Vd*sin(wt-2pi/3) + Vq*cos(wt-2pi/3) + Vo
  note: Va= Vd*sinwt + Vq*cos(wt) + Vo
  dq : Inport
  theda : Inport  Port=2
  Fcn : Fcn  Expr=(u(1)*sin(u(3))+u(2)*cos(u(3)))
  Fcn1 : Fcn  Expr=(u(1)*sin(u(3)-2*pi/3)+u(2)*cos(u(3)-2*pi/3))
  Fcn2 : Fcn  Expr=(u(1)*sin(u(3)+2*pi/3)+u(2)*cos(u(3)+2*pi/3))
  Mux1 : Mux  Inputs=2
  Mux3 : Mux  Inputs=3
  abc : Outport  VectorParamsAs1DForOutWhenUnconnected=off
  wires:
  Mux3/1 -> abc/1  "abc"
  theda/1 -> Mux1/2
  dq/1 -> Mux1/1
  Mux1/1 -> Fcn1/1, Fcn2/1, Fcn/1
  Fcn/1 -> Mux3/1
  Fcn1/1 -> Mux3/2
  Fcn2/1 -> Mux3/3

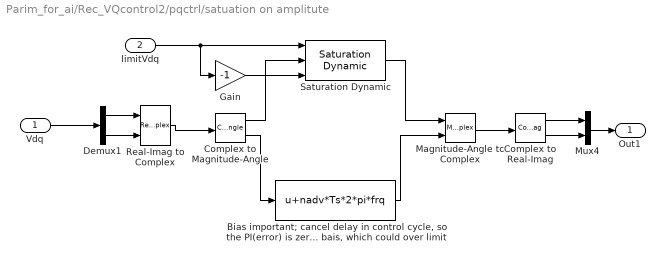
== system Parim_for_ai/Rec_VQcontrol2/pqctrl/satuation on amplitute  ==
  Vdq : Inport
  limitVdq : Inport  Port=2
  "Bias important; cancel delay in control cycle, so the PI(error) is zero, other wise PI(errer) is bais, which could over limit" : Bias  Bias=nadv*Ts*2*pi*frq  SaturateOnIntegerOverflow=off
  Complex to Magnitude-Angle : ComplexToMagnitudeAngle
  Complex to Real-Imag : ComplexToRealImag
  Demux1 : Demux  Outputs=2
  Gain : Gain  Gain=-1
  Magnitude-Angle to Complex : MagnitudeAngleToComplex
  Mux4 : Mux  Inputs=2
  Real-Imag to Complex : RealImagToComplex
  Saturation Dynamic : simulink/Discontinuities/Saturation Dynamic  OutMin=[]  OutMax=[]  OutDataTypeStr=Inherit: Same as second input  OutDataType=fixdt(1, 16)  OutScaling=2^-10  DoSatur=off
  Out1 : Outport  VectorParamsAs1DForOutWhenUnconnected=off
  wires:
  Vdq/1 -> Demux1/1
  Mux4/1 -> Out1/1
  Complex to Real-Imag/1 -> Mux4/1
  Complex to Real-Imag/2 -> Mux4/2
  Magnitude-Angle to Complex/1 -> Complex to Real-Imag/1
  Complex to Magnitude-Angle/2 -> "Bias important; cancel delay in control cycle, so the PI(error) is zero, other wise PI(errer) is bais, which could over limit"/1
  Real-Imag to Complex/1 -> Complex to Magnitude-Angle/1
  Demux1/2 -> Real-Imag to Complex/2
  Demux1/1 -> Real-Imag to Complex/1
  Saturation Dynamic/1 -> Magnitude-Angle to Complex/1
  Complex to Magnitude-Angle/1 -> Saturation Dynamic/2
  limitVdq/1 -> Gain/1, Saturation Dynamic/1
  Gain/1 -> Saturation Dynamic/3
  "Bias important; cancel delay in control cycle, so the PI(error) is zero, other wise PI(errer) is bais, which could over limit"/1 -> Magnitude-Angle to Complex/2

== system Parim_for_ai/Rec_VQcontrol8/Vdc ctrl/Vdc_ctrler1 ==
  Vcap : Inport
  Add2 : Sum  Inputs=+-
  PI_d2 : Subsystem  AncestorBlock=|  DialogController=POWERSYS.PowerSysDialog  mask(Discrete PI Controller){Kp=Kvdc(1), Ki=Kvdc(2), Par_Limits=[1 -1]*1, Init=0, Ts=Ts}
      | powerlib_extras/Discrete 
      | Control Blocks/Discrete
      | PI Controller
      mask prompts: Kp "Proportional gain (Kp):"; Ki "Integral gain (Ki):"; Par_Limits "Output limits: [ Upper   Lower ]"; Init "Output initial value:"; Ts "Sample time:"
      mask help: This block implements a discrete PI controller.
      mask init:
      | UpperLimit=Par_Limits(1);
      | LowerLimit=Par_Limits(2);
      | power_initmask();
      mask Help: This block is part of a subset of blocks in the Extras library that does not have documentation associated with it, other than the block mask description.
      mask Display: disp('PI');
  Saturation : Saturate  UpperLimit=0.1  LowerLimit=-0.1
      settings: AttributesFormatString=%<LowerLimit>~%<UpperLimit>
  Vdcpuref : Constant
  Vdctrl : Scope  NumInputPorts=2
  delP : Outport  OutputWhenDisabled=reset  InitialOutput=[0]  VectorParamsAs1DForOutWhenUnconnected=off
  wires:
  PI_d2/1(Out) -> delP/1, Vdctrl/2  "PIVdc"
  Saturation/1 -> PI_d2/1(Error)
  Vdcpuref/1 -> Add2/2
  Vcap/1 -> Add2/1, Vdctrl/1
  Add2/1 -> Saturation/1  "delVdc"

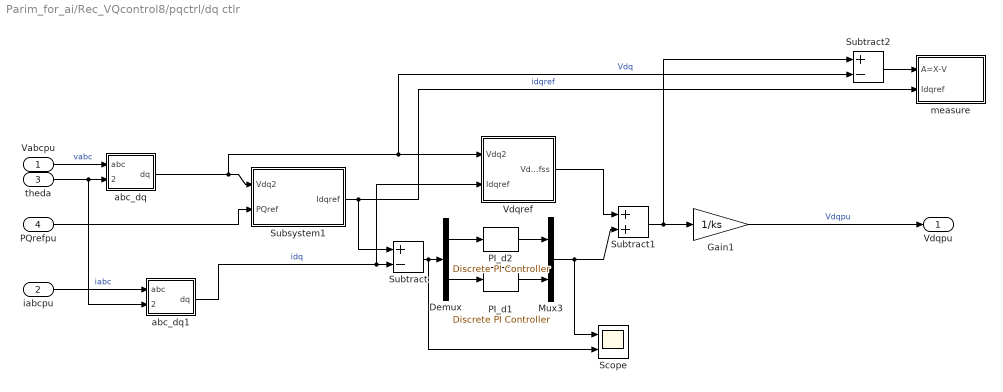
== system Parim_for_ai/Rec_VQcontrol8/pqctrl/dq ctlr ==
  Vabcpu : Inport
  iabcpu : Inport  Port=2
  theda : Inport  Port=3
  PQrefpu : Inport  Port=4
  Demux : Demux  Outputs=2
  Gain1 : Gain  Gain=1/ks
  Mux3 : Mux  Inputs=2
  PI_d1 : powerlib_extras/Discrete  Control Blocks/Discrete PI Controller  Kp=Kp(1)  Ki=Kp(2)  Par_Limits=[1 -1]*0.15  Init=0  Ts=Ts
  PI_d2 : powerlib_extras/Discrete  Control Blocks/Discrete PI Controller  Kp=Kd(1)  Ki=Kd(2)  Par_Limits=[1 -1]*0.25  Init=0  Ts=Ts
  Scope : Scope  NumInputPorts=2
  Subsystem1 : Subsystem
  Subtract : Sum  Inputs=+-
  Subtract1 : Sum
  Subtract2 : Sum  Inputs=+-
  Vdqref : Subsystem
  abc_dq : Subsystem
  abc_dq1 : Subsystem
  measure : Subsystem
  Vdqpu : Outport  VectorParamsAs1DForOutWhenUnconnected=off
  wires:
  Subtract2/1 -> measure/1(A=X-V)
  Subsystem1/1(Idqref) -> measure/2(Idqref), Subtract/1  "idqref"
  abc_dq/1(dq) -> Subtract2/2, Vdqref/1(Vdq2), Subsystem1/1(Vdq2)  "Vdq"
  abc_dq1/1(dq) -> Vdqref/2(Idqref), Subtract/2  "idq"
  Subtract/1 -> Scope/2, Demux/1
  Demux/1 -> PI_d2/1
  Demux/2 -> PI_d1/1
  Vdqref/1(Vdqrefss) -> Subtract1/1
  PI_d2/1 -> Mux3/1
  PI_d1/1 -> Mux3/2
  Mux3/1 -> Scope/1, Subtract1/2
  Subtract1/1 -> Subtract2/1, Gain1/1
  Vabcpu/1 -> abc_dq/1(abc)  "vabc"
  theda/1 -> abc_dq/2(theta), abc_dq1/2(theta)
  PQrefpu/1 -> Subsystem1/2(PQref)
  iabcpu/1 -> abc_dq1/1(abc)  "iabc"
  Gain1/1 -> Vdqpu/1  "Vdqpu"

== system Parim_for_ai/Rec_VQcontrol8/pqctrl/dq->abc ==
  note: Va= Vd*sinwt + Vq*cos(wt) + Vo
  note: Vb= Vd*sin(wt-2pi/3) + Vq*cos(wt-2pi/3) + Vo
  note: Vc= Vd*sin(wt+2pi/3) + Vq*cos(wt+2pi/3) + Vo
  dq : Inport
  theda : Inport  Port=2
  Fcn : Fcn  Expr=(u(1)*sin(u(3))+u(2)*cos(u(3)))
  Fcn1 : Fcn  Expr=(u(1)*sin(u(3)-2*pi/3)+u(2)*cos(u(3)-2*pi/3))
  Fcn2 : Fcn  Expr=(u(1)*sin(u(3)+2*pi/3)+u(2)*cos(u(3)+2*pi/3))
  Mux1 : Mux  Inputs=2
  Mux3 : Mux  Inputs=3
  abc : Outport  VectorParamsAs1DForOutWhenUnconnected=off
  wires:
  Fcn2/1 -> Mux3/3
  Fcn1/1 -> Mux3/2
  Fcn/1 -> Mux3/1
  Mux1/1 -> Fcn/1, Fcn2/1, Fcn1/1
  dq/1 -> Mux1/1
  theda/1 -> Mux1/2
  Mux3/1 -> abc/1  "abc"

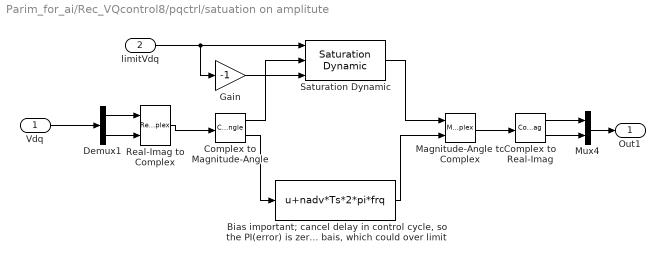
== system Parim_for_ai/Rec_VQcontrol8/pqctrl/satuation on amplitute  ==
  Vdq : Inport
  limitVdq : Inport  Port=2
  "Bias important; cancel delay in control cycle, so the PI(error) is zero, other wise PI(errer) is bais, which could over limit" : Bias  Bias=nadv*Ts*2*pi*frq  SaturateOnIntegerOverflow=off
  Complex to Magnitude-Angle : ComplexToMagnitudeAngle
  Complex to Real-Imag : ComplexToRealImag
  Demux1 : Demux  Outputs=2
  Gain : Gain  Gain=-1
  Magnitude-Angle to Complex : MagnitudeAngleToComplex
  Mux4 : Mux  Inputs=2
  Real-Imag to Complex : RealImagToComplex
  Saturation Dynamic : simulink/Discontinuities/Saturation Dynamic  OutMin=[]  OutMax=[]  OutDataTypeStr=Inherit: Same as second input  OutDataType=fixdt(1, 16)  OutScaling=2^-10  DoSatur=off
  Out1 : Outport  VectorParamsAs1DForOutWhenUnconnected=off
  wires:
  "Bias important; cancel delay in control cycle, so the PI(error) is zero, other wise PI(errer) is bais, which could over limit"/1 -> Magnitude-Angle to Complex/2
  Gain/1 -> Saturation Dynamic/3
  limitVdq/1 -> Saturation Dynamic/1, Gain/1
  Complex to Magnitude-Angle/1 -> Saturation Dynamic/2
  Saturation Dynamic/1 -> Magnitude-Angle to Complex/1
  Demux1/1 -> Real-Imag to Complex/1
  Demux1/2 -> Real-Imag to Complex/2
  Real-Imag to Complex/1 -> Complex to Magnitude-Angle/1
  Complex to Magnitude-Angle/2 -> "Bias important; cancel delay in control cycle, so the PI(error) is zero, other wise PI(errer) is bais, which could over limit"/1
  Magnitude-Angle to Complex/1 -> Complex to Real-Imag/1
  Complex to Real-Imag/2 -> Mux4/2
  Complex to Real-Imag/1 -> Mux4/1
  Mux4/1 -> Out1/1
  Vdq/1 -> Demux1/1

== system Parim_for_ai/Rec_VQcontrol2/Vdc ctrl/Vdc_ctrler1/PI_d2 ==
  note: Pierre Giroux, Gilbert Sybille
      | Power System Simulation Laboratory
      | IREQ, Hydro-Quebc
  note: Discrete PID Controller
  Error : Inport  SampleTime=Ts
  Discrete-Time Integrator : DiscreteIntegrator  InitialCondition=Init  SampleTime=Ts  LimitOutput=on  UpperSaturationLimit=UpperLimit  LowerSaturationLimit=LowerLimit  ICPrevOutput=DiscIntNeverNeededParam  ICPrevScaledInput=DiscIntNeverNeededParam
  Kp4 : Gain  Gain=Kp  SaturateOnIntegerOverflow=on  SampleTime=Ts  OutDataTypeStr=Inherit: Same as input  ParamDataTypeStr=Inherit: Same as input
  Kp5 : Gain  Gain=Ki  SaturateOnIntegerOverflow=on  SampleTime=Ts  OutDataTypeStr=Inherit: Same as input  ParamDataTypeStr=Inherit: Same as input
  Saturation2 : Saturate  UpperLimit=UpperLimit  LowerLimit=LowerLimit  SampleTime=Ts
  Sum6 : Sum  InputSameDT=on  SaturateOnIntegerOverflow=on  SampleTime=Ts  OutDataTypeStr=Inherit: Same as first input
  Zero-Order Hold : ZeroOrderHold  SampleTime=Ts
  Out : Outport  SampleTime=Ts  InitialOutput=0  VectorParamsAs1DForOutWhenUnconnected=off
  wires:
  Error/1 -> Kp4/1, Kp5/1
  Sum6/1 -> Saturation2/1
  Kp5/1 -> Discrete-Time Integrator/1
  Kp4/1 -> Zero-Order Hold/1
  Discrete-Time Integrator/1 -> Sum6/2  "int"
  Saturation2/1 -> Out/1
  Zero-Order Hold/1 -> Sum6/1  "prop"

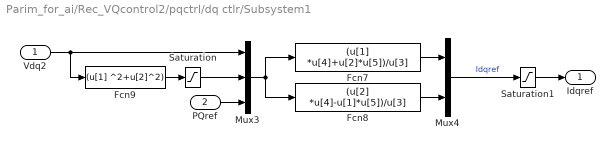
== system Parim_for_ai/Rec_VQcontrol2/pqctrl/dq ctlr/Subsystem1 ==
  Vdq2 : Inport
  PQref : Inport  Port=2
  Fcn7 : Fcn  Expr=(u[1] *u[4]+u[2]*u[5])/u[3]
  Fcn8 : Fcn  Expr=(u[2] *u[4]-u[1]*u[5])/u[3]
  Fcn9 : Fcn  Expr=(u[1] ^2+u[2]^2)
  Mux3 : Mux  Inputs=[2 1 2]
  Mux4 : Mux  Inputs=2
  Saturation : Saturate  UpperLimit=inf  LowerLimit=0.01
  Saturation1 : Saturate  UpperLimit=1.5  LowerLimit=-1.5
  Idqref : Outport  VectorParamsAs1DForOutWhenUnconnected=off
  wires:
  Saturation/1 -> Mux3/2
  PQref/1 -> Mux3/3
  Mux4/1 -> Saturation1/1  "Idqref"
  Fcn8/1 -> Mux4/2
  Fcn7/1 -> Mux4/1
  Fcn9/1 -> Saturation/1
  Mux3/1 -> Fcn7/1, Fcn8/1
  Vdq2/1 -> Mux3/1, Fcn9/1
  Saturation1/1 -> Idqref/1

== system Parim_for_ai/Rec_VQcontrol2/pqctrl/dq ctlr/Vdqref ==
  Vdq2 : Inport
  Idqref : Inport  Port=2
  Display : Display
      settings: Decimation=50
  Fcn7 : Fcn  Expr=(u[2] +u[4]*u[5]+u[3]*u[6])
  Fcn8 : Fcn  Expr=(u[1] +u[3]*u[5]-u[4]*u[6])
  Lxpu : Constant  Value=Lxpu
  Mux3 : Mux
  Mux4 : Mux  Inputs=2
  Rxpu : Constant  Value=Rxpu
  Vdqrefss : Outport  VectorParamsAs1DForOutWhenUnconnected=off
  wires:
  Mux4/1 -> Vdqrefss/1
  Idqref/1 -> Mux3/2
  Vdq2/1 -> Mux3/1
  Fcn7/1 -> Mux4/2  "Vqref"
  Fcn8/1 -> Mux4/1  "Vdref"
  Mux3/1 -> Fcn7/1, Fcn8/1, Display/1
  Rxpu/1 -> Mux3/3
  Lxpu/1 -> Mux3/4
